simulink model "speedControl_BLDCmotor"  (R2020a)
settings: Solver=VariableStepAuto  StartTime=0.0  StopTime=10.0  RelTol=1e-3
libraries: simulink x1
settings Model: Creator=DELL  LastModifiedBy=DELL

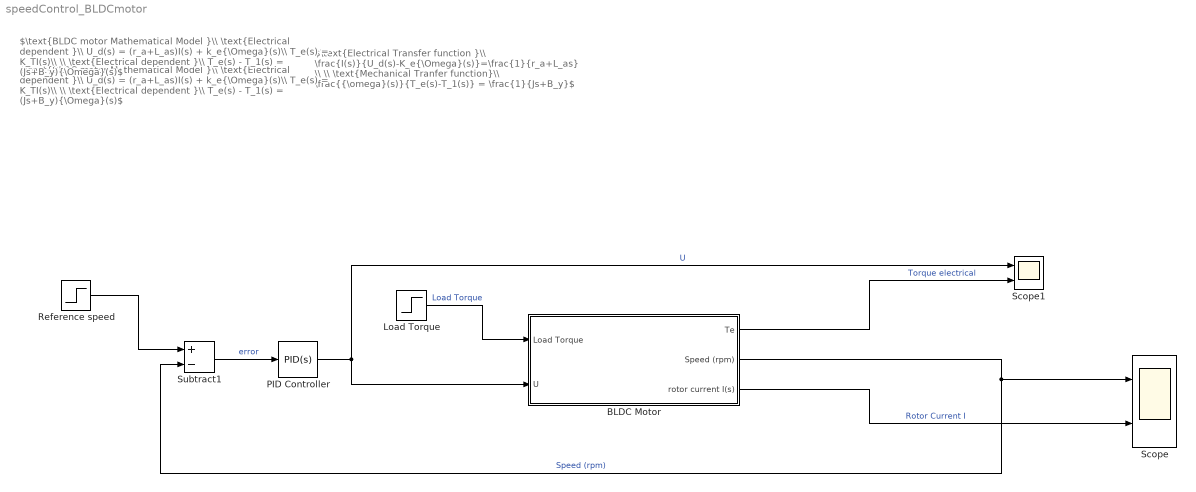
== system speedControl_BLDCmotor ==
  note: $\text{Electrical Transfer function }\\ \frac{I(s)}{U_d(s)-K_e{\Omega}(s)}=\frac{1}{r_a+L_as} \\ \\ \text{Mechanical Tranfer function}\\ \frac{{\omega}(s)}{T_e(s)-T_1(s)} = \frac{1}{Js+B_y}$
  note: $\text{BLDC motor Mathematical Model }\\ \text{Electrical dependent }\\ U_d(s) = (r_a+L_as)I(s) + k_e{\Omega}(s)\\ T_e(s) = K_TI(s)\\ \\ \text{Electrical dependent }\\ T_e(s) - T_1(s) = (Js+B_y){\Omega}(s)$
  note: $\text{BLDC motor Mathematical Model }\\ \text{Electrical dependent }\\ U_d(s) = (r_a+L_as)I(s) + k_e{\Omega}(s)\\ T_e(s) = K_TI(s)\\ \\ \text{Electrical dependent }\\ T_e(s) - T_1(s) = (Js+B_y){\Omega}(s)$
  BLDC Motor : Subsystem  mask{La=0.1e-3, ra=0.013, J=0.0045, By=0.01, Kt=0.15, Ke=0.19}
      mask prompts: La "Winding Inductance (La)"; ra "Winding Resistance (ra)"; J "Movement of Intertia (J)"; By "Coefficient of viscous friction (By)"; Kt "Torque Constant (Kt)"; Ke "Back emf Constant (Ke)"
      mask DialogControl DescGroupVar Prompt: BLDC Motor
      mask DialogControl DescTextVar Prompt: Brushless DC Motor Parameters
      mask DialogControl Container4 Prompt: Electrical Parameters
      mask DialogControl Container6 Prompt: Mechanical Parameters
      mask DialogControl Container10 Prompt: Constant Gains
  Load Torque : Step  Time=2  SampleTime=0
  PID Controller : simulink/Continuous/PID Controller  Controller=PID  Form=Parallel  TimeDomain=Continuous-time  UseExternalTs=off  SampleTime=-1  IntegratorMethod=Forward Euler  FilterMethod=Forward Euler  ControllerParametersSource=internal  P=0.00556186665025774  I=0.49368871899943  D=1.54848512733453e-05  UseFilter=on  N=37950.487723144  TunerSelectOption=Transfer Function Based (PID Tuner App)  InitialConditionSource=internal  InitialConditionForIntegrator=0  InitialConditionForFilter=0  DifferentiatorICPrevScaledInput=0  ExternalReset=none  TrackingMode=off  Kt=1  LimitOutput=off  UpperSaturationLimit=inf  LowerSaturationLimit=-inf  LinearizeAsGain=on  AntiWindupMode=none  Kb=1  POutMin=[]  POutMax=[]  IOutMin=[]  IOutMax=[]  DOutMin=[]  DOutMax=[]  NOutMin=[]  NOutMax=[]  SumOutMin=[]  SumOutMax=[]  SaturationOutMin=[]  SaturationOutMax=[]  PParamMin=[]  PParamMax=[]  IParamMin=[]  IParamMax=[]  DParamMin=[]  DParamMax=[]  NParamMin=[]  NParamMax=[]  KbParamMin=[]  KbParamMax=[]  KtParamMin=[]  KtParamMax=[]  KbOutMin=[]  KbOutMax=[]  KtOutMin=[]  KtOutMax=[]  IntegratorOutMin=[]  IntegratorOutMax=[]  FilterOutMin=[]  FilterOutMax=[]  SumI1OutMin=[]  SumI1OutMax=[]  SumI2OutMin=[]  SumI2OutMax=[]  SumI3OutMin=[]  SumI3OutMax=[]  SumI4OutMin=[]  SumI4OutMax=[]  SumDOutMin=[]  SumDOutMax=[]  DifferentiatorOutMin=[]  DifferentiatorOutMax=[]  FilterDiffOutCoefMin=[]  FilterDiffOutCoefMax=[]  ReciprocalOutMin=[]  ReciprocalOutMax=[]  SumDenOutMin=[]  SumDenOutMax=[]  SumNumOutMin=[]  SumNumOutMax=[]  DivideOutMin=[]  DivideOutMax=[]  UdiffTsProdOutMin=[]  UdiffTsProdOutMax=[]  NTsProdOutMin=[]  NTsProdOutMax=[]  UintegralTsProdOutMin=[]  UintegralTsProdOutMax=[]  UngainTsProdOutMin=[]  UngainTsProdOutMax=[]  IntegratorContinuousStateAttributes=''  IntegratorStateMustResolveToSignalObject=off  IntegratorRTWStateStorageClass=Auto  FilterContinuousStateAttributes=''  FilterStateMustResolveToSignalObject=off  FilterRTWStateStorageClass=Auto  ParallelPVariant=InternalParameters  IdealPVariant=Disabled  IVariant=InternalParameters  DVariant=InternalParameters  IntegratorVariant=Continuous  SatVariant=Disabled  AWVariant=Passthrough  PCopyVariant=Disabled  TRVariant=Disabled  FdbkBlocksVariant=Forward  IdealPFdbkVariant=Disabled  SatFdbkVariant=Disabled  DerivativeFilterVariant=ContFilter  NVariant=InternalParameters  NCopyVariant=Disabled  FilterICVariant=InternalICsFilter  IntegratorICVariant=InternalICs  ExternalResetVariant=Disabled  TRSumVariant=Passthrough  SumFdbkVariant=Disabled  SumVariant=Sum_PID  TsampFilterVariant=InternalTs  TsampNgainVariant=Passthrough  TsampIntegralVariant=Passthrough
  Reference speed : Step  After=60  SampleTime=0
  Scope : Scope  NumInputPorts=2
  Scope1 : Scope  NumInputPorts=2
  Subtract1 : Sum  Inputs=+-
  wires:
  PID Controller/1 -> BLDC Motor/2(U), Scope1/1  "U"
  Subtract1/1 -> PID Controller/1  "error"
  Reference speed/1 -> Subtract1/1
  BLDC Motor/2(Speed (rpm)) -> Subtract1/2, Scope/1  "Speed (rpm)"
  Load Torque/1 -> BLDC Motor/1(Load Torque)  "Load Torque"
  BLDC Motor/1(Te) -> Scope1/2  "Torque electrical"
  BLDC Motor/3(rotor current I(s)) -> Scope/2  "Rotor Current I"

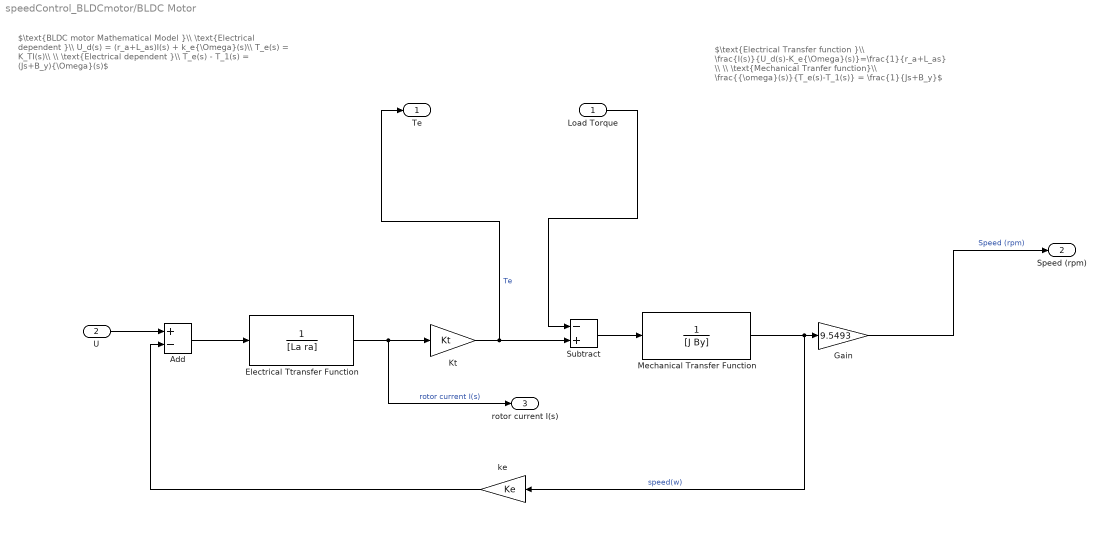
== system speedControl_BLDCmotor/BLDC Motor ==
  note: $\text{Electrical Transfer function }\\ \frac{I(s)}{U_d(s)-K_e{\Omega}(s)}=\frac{1}{r_a+L_as} \\ \\ \text{Mechanical Tranfer function}\\ \frac{{\omega}(s)}{T_e(s)-T_1(s)} = \frac{1}{Js+B_y}$
  note: $\text{BLDC motor Mathematical Model }\\ \text{Electrical dependent }\\ U_d(s) = (r_a+L_as)I(s) + k_e{\Omega}(s)\\ T_e(s) = K_TI(s)\\ \\ \text{Electrical dependent }\\ T_e(s) - T_1(s) = (Js+B_y){\Omega}(s)$
  Load Torque : Inport
  U : Inport  Port=2
  Add : Sum  Inputs=+-
  Electrical Ttransfer Function : TransferFcn  Denominator=[La ra]
  Gain : Gain  Gain=9.5493
  Kt : Gain  Gain=Kt
  Mechanical Transfer Function : TransferFcn  Denominator=[J By]
  Subtract : Sum  Inputs=-+
  ke : Gain  Gain=Ke
  Te : Outport
  Speed (rpm) : Outport  Port=2
  rotor current I(s) : Outport  Port=3
  wires:
  Electrical Ttransfer Function/1 -> rotor current I(s)/1, Kt/1  "rotor current I(s)"
  Kt/1 -> Te/1, Subtract/2  "Te"
  ke/1 -> Add/2
  Gain/1 -> Speed (rpm)/1  "Speed (rpm)"
  Mechanical Transfer Function/1 -> ke/1, Gain/1  "speed(w)"
  Load Torque/1 -> Subtract/1
  Add/1 -> Electrical Ttransfer Function/1
  Subtract/1 -> Mechanical Transfer Function/1
  U/1 -> Add/1
